simulink model "position_control"  (R2024a)
settings: Solver=VariableStepAuto  StartTime=0.0  StopTime=60  MaxStep=0.1  RelTol=1e-3
values from neighbouring files (symbols this model uses):
  F_max = 50    [init.m]
  F_min = -50    [init.m]
  k = 0.5    [init.m]
  kbc = 0.05    [init.m]
  kd = 2    [init.m]
  ki = 2    [init.m]
  kp = 20    [init.m]
  m = 10    [init.m]
  tau = 0.1    [init.m]
settings Model: Creator=berto  LastModifiedBy=berto

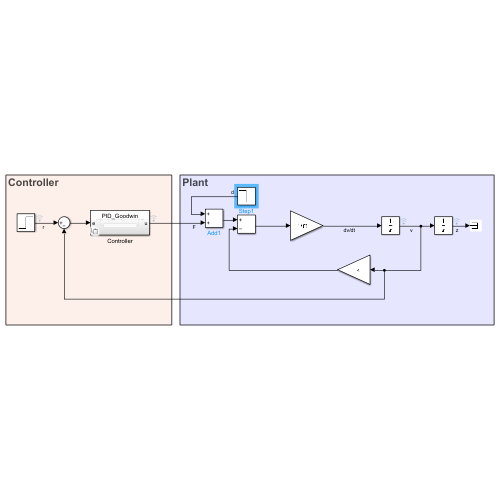
[thumbnail: Simulink's stored preview of the top-level diagram]
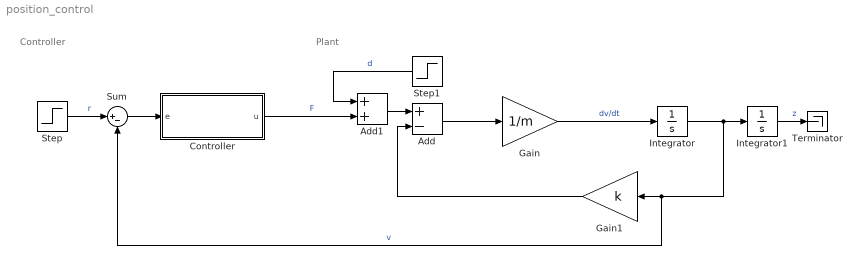
== system position_control ==
  note: Controller
  note: Plant
  Add : Sum  Inputs=+-
  Add1 : Sum
  Controller : Subsystem  Variant=on
  Gain : Gain  Gain=1/m
  Gain1 : Gain  Gain=k
  Integrator : Integrator
  Integrator1 : Integrator
  Step : Step  After=20  SampleTime=0
  Step1 : Step  Time=30  After=-30  SampleTime=0
  Sum : Sum  Inputs=|+-
  Terminator : Terminator
  wires:
  Controller/1(u) -> Add1/2  "F"
  Step/1 -> Sum/1  "r"
  Sum/1 -> Controller/1(e)
  Add/1 -> Gain/1
  Gain/1 -> Integrator/1  "dv/dt"
  Integrator/1 -> Sum/2, Gain1/1, Integrator1/1  "v"
  Gain1/1 -> Add/2
  Step1/1 -> Add1/1  "d"
  Add1/1 -> Add/1
  Integrator1/1 -> Terminator/1  "z"

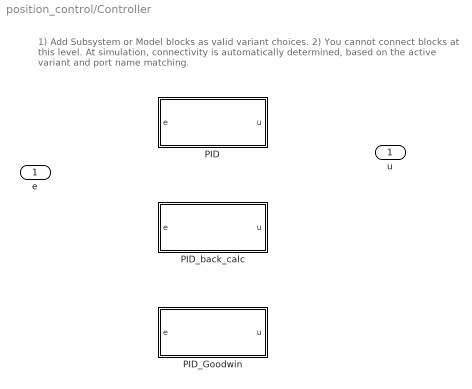
== system position_control/Controller ==
  note: 1) Add Subsystem or Model blocks as valid variant choices.
      | 2) You cannot connect blocks at this level. At simulation, connectivity is automatically
      | determined, based on the active variant and port name matching.
  e : Inport
  PID : Subsystem  VariantControl=ctrl_type == 0
  PID_Goodwin : Subsystem  VariantControl=ctrl_type == 2
  PID_back_calc : Subsystem  VariantControl=ctrl_type == 1
  u : Outport

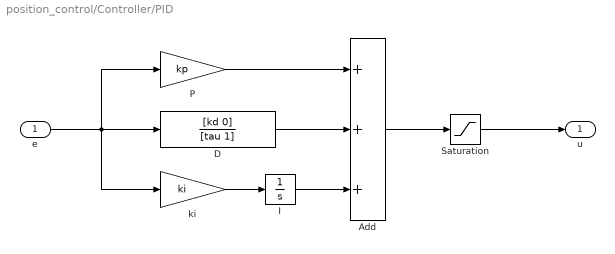
== system position_control/Controller/PID ==
  e : Inport
  Add : Sum  Inputs=+++
  D : TransferFcn  Numerator=[kd 0]  Denominator=[tau 1]
  I : Integrator
  P : Gain  Gain=kp
  Saturation : Saturate  UpperLimit=F_max  LowerLimit=F_min
  ki : Gain  Gain=ki
  u : Outport
  wires:
  ki/1 -> I/1
  Add/1 -> Saturation/1
  D/1 -> Add/2
  I/1 -> Add/3
  P/1 -> Add/1
  e/1 -> ki/1, P/1, D/1
  Saturation/1 -> u/1

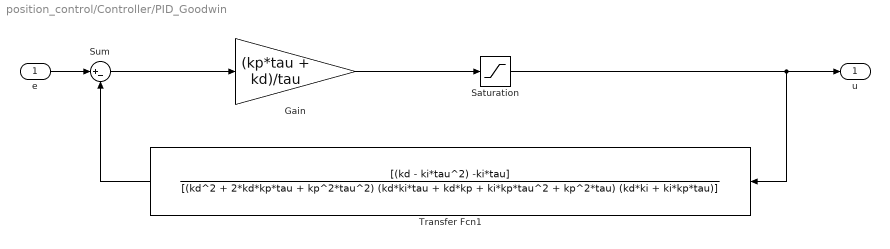
== system position_control/Controller/PID_Goodwin ==
  e : Inport
  Gain : Gain  Gain=(kp*tau + kd)/tau
  Saturation : Saturate  UpperLimit=F_max  LowerLimit=F_min
  Sum : Sum  Inputs=|+-
  Transfer Fcn1 : TransferFcn  Numerator=[(kd - ki*tau^2) -ki*tau]  Denominator=[(kd^2 + 2*kd*kp*tau + kp^2*tau^2) (kd*ki*tau + kd*kp + ki*kp*tau^2 + kp^2*tau) (kd*ki + ki*kp*tau)]
  u : Outport
  wires:
  e/1 -> Sum/1
  Saturation/1 -> Transfer Fcn1/1, u/1
  Sum/1 -> Gain/1
  Gain/1 -> Saturation/1
  Transfer Fcn1/1 -> Sum/2

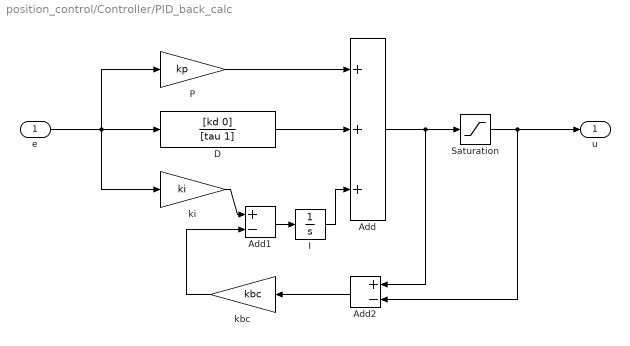
== system position_control/Controller/PID_back_calc ==
  e : Inport
  Add : Sum  Inputs=+++
  Add1 : Sum  Inputs=+-
  Add2 : Sum  Inputs=+-
  D : TransferFcn  Numerator=[kd 0]  Denominator=[tau 1]
  I : Integrator
  P : Gain  Gain=kp
  Saturation : Saturate  UpperLimit=F_max  LowerLimit=F_min
  kbc : Gain  Gain=kbc
  ki : Gain  Gain=ki
  u : Outport
  wires:
  Add/1 -> Add2/1, Saturation/1
  e/1 -> ki/1, P/1, D/1
  D/1 -> Add/2
  P/1 -> Add/1
  Saturation/1 -> Add2/2, u/1
  Add1/1 -> I/1
  ki/1 -> Add1/1
  kbc/1 -> Add1/2
  Add2/1 -> kbc/1
  I/1 -> Add/3
